simulink model "RegimePermanente"  (Simulink 7.1)
settings: Solver=ode45  StartTime=0.0  StopTime=10.0  RelTol=1e-3
settings Model: Creator=George  LastModifiedBy=George

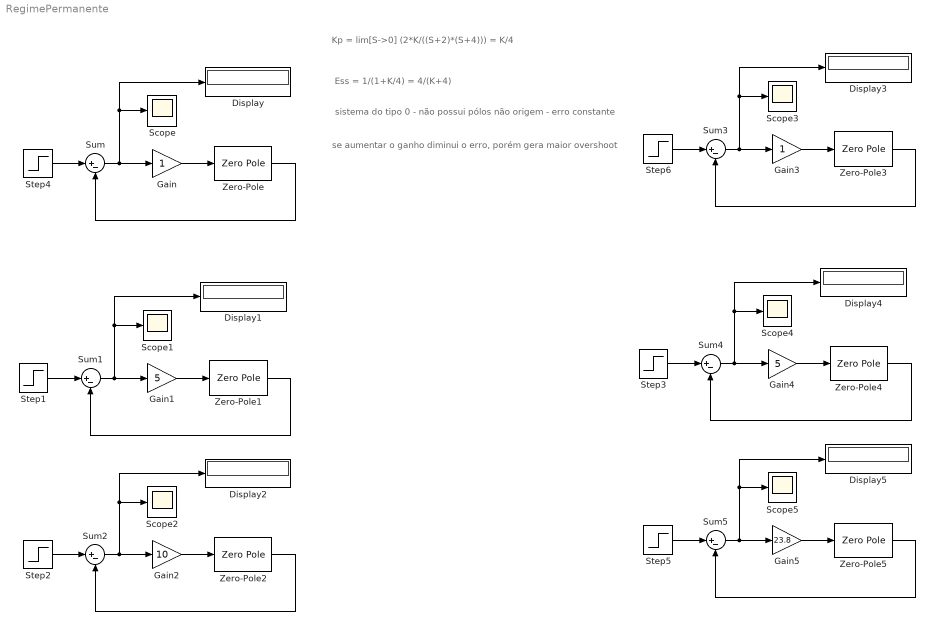
== system RegimePermanente ==
  note: Kp = lim[S->0] (2*K/((S+2)*(S+4))) = K/4
  note: Ess = 1/(1+K/4) = 4/(K+4)
  note: sistema do tipo 0 - não possui pólos não origem - erro constante
  note: se aumentar o ganho diminui o erro, porém gera maior overshoot
  Display{,1..5} (6 alike) : Display
  Gain : Gain  ParameterDataType=sfix(16)  ParameterScaling=2^0  OutDataType=sfix(16)  OutScaling=2^0
  Gain1 : Gain  Gain=5  ParameterDataType=sfix(16)  ParameterScaling=2^0  OutDataType=sfix(16)  OutScaling=2^0
  Gain2 : Gain  Gain=10  ParameterDataType=sfix(16)  ParameterScaling=2^0  OutDataType=sfix(16)  OutScaling=2^0
  Gain3 : Gain  ParameterDataType=sfix(16)  ParameterScaling=2^0  OutDataType=sfix(16)  OutScaling=2^0
  Gain4 : Gain  Gain=5  ParameterDataType=sfix(16)  ParameterScaling=2^0  OutDataType=sfix(16)  OutScaling=2^0
  Gain5 : Gain  Gain=23.8  ParameterDataType=sfix(16)  ParameterScaling=2^0  OutDataType=sfix(16)  OutScaling=2^0
  Scope{,1..5} (6 alike) : Scope
      Scope2 settings: SaveName=ScopeData2
      Scope3 settings: SaveName=ScopeData3
      Scope4 settings: SaveName=ScopeData4
      Scope5 settings: SaveName=ScopeData5
  Step{1..6} (6 alike) : Step  Time=0  SampleTime=0
  Sum{,1..5} (6 alike) : Sum  Inputs=|+-  OutDataType=sfix(16)  OutScaling=2^0
  Zero-Pole : ZeroPole  Zeros=[]  Poles=[-2 -4]  Gain=2
  Zero-Pole1 : ZeroPole  Zeros=[]  Poles=[-2 -4]  Gain=2
  Zero-Pole2 : ZeroPole  Zeros=[]  Poles=[-2 -4]  Gain=2
  Zero-Pole3 : ZeroPole  Zeros=[]  Poles=[-2 -4 0]  Gain=2
  Zero-Pole4 : ZeroPole  Zeros=[]  Poles=[-2 -4 0]  Gain=2
  Zero-Pole5 : ZeroPole  Zeros=[]  Poles=[-2 -4 0]  Gain=2
  wires:
  Sum/1 -> Gain/1, Scope/1, Display/1
  Gain/1 -> Zero-Pole/1
  Zero-Pole/1 -> Sum/2
  Step4/1 -> Sum/1
  Sum1/1 -> Gain1/1, Scope1/1, Display1/1
  Gain1/1 -> Zero-Pole1/1
  Zero-Pole1/1 -> Sum1/2
  Step1/1 -> Sum1/1
  Sum2/1 -> Gain2/1, Scope2/1, Display2/1
  Gain2/1 -> Zero-Pole2/1
  Zero-Pole2/1 -> Sum2/2
  Step2/1 -> Sum2/1
  Sum3/1 -> Gain3/1, Scope3/1, Display3/1
  Gain3/1 -> Zero-Pole3/1
  Zero-Pole3/1 -> Sum3/2
  Step6/1 -> Sum3/1
  Sum4/1 -> Gain4/1, Scope4/1, Display4/1
  Gain4/1 -> Zero-Pole4/1
  Zero-Pole4/1 -> Sum4/2
  Step3/1 -> Sum4/1
  Sum5/1 -> Gain5/1, Scope5/1, Display5/1
  Gain5/1 -> Zero-Pole5/1
  Zero-Pole5/1 -> Sum5/2
  Step5/1 -> Sum5/1
